simulink model "mcb_pmsm_foc_sensorless_f28379d1"  (R2026a)
settings: Solver=FixedStepDiscrete  StopTime=8  EnableMultiTasking=on
InitFcn:
  | mcb_pmsm_foc_sensorless_f28379d_datascript; mcb_pmsm_foc_sensorless_f28379d_kre_setup; mcb_pmsm_foc_sensorless_f28379d_spmsm_based_ipmsm_setup;
model workspace (MAT data in the model file):
  encoderResolution = 2000
  hallOffset = '0.5'
  indexOffset = 850
  polePairs = '4'
values from neighbouring files (symbols this model uses):
  acceleration = 10000/PU_System.N_base    [mcb_pmsm_foc_sensorless_f28379d_datascript.m]
  dataType = 'single'    [mcb_pmsm_foc_sensorless_f28379d_datascript.m]
  inverter = mcb.updateInverterParameters(pmsm,inverter,target)    [mcb_pmsm_foc_sensorless_f28379d_datascript.m]    (also in mcb_pmsm_foc_sensorless_f28379d_kre_setup.m = inverterSPMSM)
  KRE_Params_Vector = single([      KRE_OBSERVER_R_RATIO * motor.Rs;      pmsm.Ld;      pmsm.Lq;      pmsm.FluxPM;      Ts;      PU_System.V_base;      PU_System.I_base;      pmsm.N_base;      pmsm.p;      KRE_Profile.Alpha;      KRE_Profile.A;      KRE_Profile.Gamma;      KRE_Profile.SigmaEpsilon;      KRE_Profile.SpeedFilterHz])    [mcb_pmsm_foc_sensorless_f28379d_kre_setup.m]
  MAX_OL_NEG_SPD = -0.2    [mcb_pmsm_foc_sensorless_f28379d_datascript.m]
  MAX_OL_POS_SPD = 0.2    [mcb_pmsm_foc_sensorless_f28379d_datascript.m]
  MAX_OL_VD_LIMIT = 0.6    [mcb_pmsm_foc_sensorless_f28379d_datascript.m]
  MIN_CL_NEG_SPD = -0.15    [mcb_pmsm_foc_sensorless_f28379d_datascript.m]
  MIN_CL_POS_SPD = 0.15    [mcb_pmsm_foc_sensorless_f28379d_datascript.m]
  MIN_OL_VD_LIMIT = 0.15    [mcb_pmsm_foc_sensorless_f28379d_datascript.m]
  one_sec_tick = uint16(1/Ts_speed)    [mcb_pmsm_foc_sensorless_f28379d_datascript.m]
  PI_params = mcb.calcFOCGains(motor,Ts,Ts_speed,Base=PU_System,PositionObserver=EEMF,SLFeedbackPathDelay=EEMFSLDelay)    [mcb_pmsm_foc_sensorless_f28379d_datascript.m]    (also in mcb_pmsm_foc_sensorless_f28379d_kre_setup.m = PI_paramsSPMSM)
  pmsm = mcb.getPMSMParameters('Teknic2310P')    [mcb_pmsm_foc_sensorless_f28379d_datascript.m]    (also in mcb_pmsm_foc_sensorless_f28379d_kre_setup.m = pmsmSPMSM)
  PU_System = mcb.getPUSystemParameters(pmsm,inverter)    [mcb_pmsm_foc_sensorless_f28379d_datascript.m]    (also in mcb_pmsm_foc_sensorless_f28379d_kre_setup.m = PU_SystemSPMSM)
  RAMP_STEP_SIZE = 0.001    [mcb_pmsm_foc_sensorless_f28379d_datascript.m]
  Speed_openLoop_PU = 0.1    [mcb_pmsm_foc_sensorless_f28379d_datascript.m]
  target = mcb.getProcessorParameters('F28379D',PWM_frequency)    [mcb_pmsm_foc_sensorless_f28379d_datascript.m]
  Ts = T_pwm    (= 5e-05)    [mcb_pmsm_foc_sensorless_f28379d_datascript.m]
  Ts_motor = T_pwm/2    (= 2.5e-05)    [mcb_pmsm_foc_sensorless_f28379d_datascript.m]
  Ts_simulink = T_pwm/2    (= 2.5e-05)    [mcb_pmsm_foc_sensorless_f28379d_datascript.m]
  Ts_speed = 10*Ts    (= 0.0005)    [mcb_pmsm_foc_sensorless_f28379d_datascript.m]
  two_sec_tick = uint16(2/Ts_speed)    [mcb_pmsm_foc_sensorless_f28379d_datascript.m]
undefined symbols (not defined in the file or in its folder): bit, DiscIntNeverNeededParam, Down, GPTRIP1SEL, GPTRIP2SEL, TZ1, TZ2, Up
libraries: mcbcontrolslib x9, c2802xlib x7, mcbeeMathTransformLib x6, simulink x6, c280xlib x5, c2837xDlib x4, slpidlib x3, mcbpositiondecoderlib x3, mcbsensorlessestimatorlib x2, svdschedulerlib x2, svdutilitieslib x1, mcbplantlib x1
(part 1 of 3)
settings Model: ExtModeTrigDuration=8  Creator=The MathWorks, Inc.  LastModifiedBy=hzldx
settings OptimizationCC: DefaultUnderspecifiedDataType=single  OptimizeBlockIOStorage=off  BufferReuse=off  GlobalBufferReuse=off  ExpressionFolding=off  LocalBlockOutputs=off  InitFltsAndDblsToZero=on  NoFixptDivByZeroProtection=on  EfficientFloat2IntCast=on  EfficientMapNaN2IntZero=off  LifeSpan=Inf  MaxStackSize=1024  OptimizeDataStoreBuffers=off  BusAssignmentInplaceUpdate=off  DenormalBehavior=FlushToZero
settings DebuggingCC: ReadBeforeWriteMsg=DisableAll  WriteAfterWriteMsg=DisableAll  WriteAfterReadMsg=DisableAll  CheckSSInitialOutputMsg=off  InheritedTsInSrcMsg=none  MultiTaskDSMMsg=none  MultiTaskCondExecSysMsg=none  TasksWithSamePriorityMsg=none  SigSpecEnsureSampleTimeMsg=none  IntegerOverflowMsg=none  ParameterPrecisionLossMsg=none  SubsystemReferenceDiagnosticForUnitTest=warning  IntegerSaturationMsg=none
settings HardwareCC: ProdBitPerChar=16.0  ProdBitPerInt=16.0  ProdLargestAtomicInteger=Integer  ProdWordSize=16.0  ProdHWDeviceType=Texas Instruments->C2000  TargetBitPerChar=16.0  TargetBitPerInt=16.0  TargetBitPerPointer=16.0  TargetLargestAtomicInteger=Integer  TargetIntDivRoundTo=Zero  TargetEndianess=LittleEndian  TargetWordSize=16.0  TargetHWDeviceType=TI C2000
settings RTWCC: SystemTargetFile=ert.tlc  HardwareBoard=TI Delfino F28379D LaunchPad  GenerateReport=on  Toolchain=Texas Instruments Code Composer Studio (C2000)  IncludeHyperlinkInReport=on  LaunchReport=on  GenerateTraceInfo=on  GenerateTraceReport=on  GenerateTraceReportSl=on  GenerateTraceReportSf=on  GenerateTraceReportEml=on  Description=Embedded Coder
settings CodeAppCC: CustomSymbolStrType=$N$R$M  InternalIdentifier=Classic
settings ERTTargetCC: ExtModeStaticAllocSize=10000.0  MemSecPackage=tic2000demospkg  DynamicArrayContainerType=coder::array  CodeReplacementLibrary=TI C28x  MultiwordLength=2048.0
settings SimscapeCC: SimscapeNominalValues="[{\"value\":\"1\",\"unit\":\"A\"},{\"value\":\"1\",\"unit\":\"bar\"},{\"value\":\"1\",\"unit\":\"cm^2\"},{\"value\":\"1\",\"unit\":\"cm^3/s\"},{\"value\":\"1\",\"unit\":\"kJ/kg\"},{\"value\":\"1\",\"unit\":\"kW\"},{\"value\":\"1\",\"unit\":\"l\"},{\"value\":\"1\",\"unit\":\"N\"},{\"value\":\"1\",\"unit\":\"N*m\"},{\"value\":\"1\",\"unit\":\"V\"}]"  SimscapeLogType=none  SimscapeLogDataHistory=5000.0

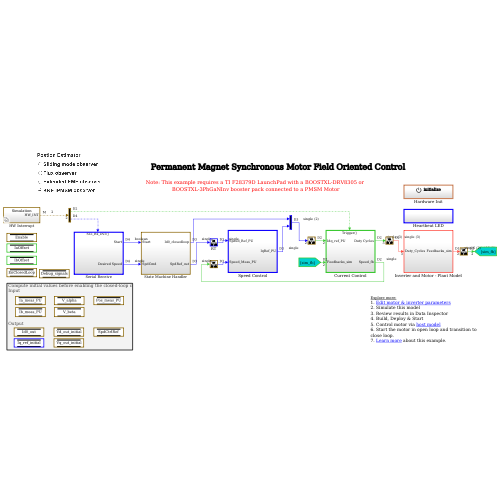
[thumbnail: Simulink's stored preview of the top-level diagram]
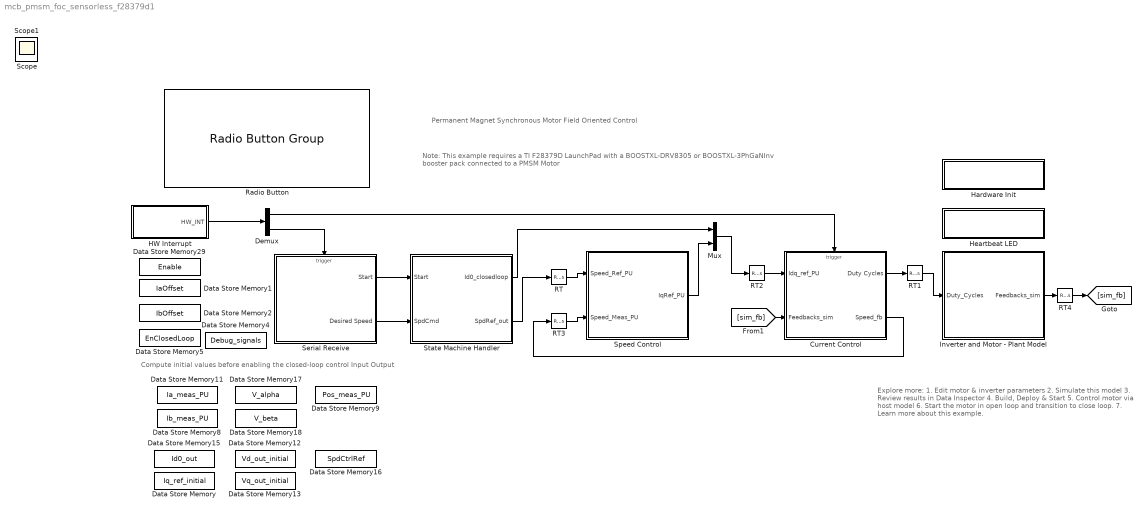
== system mcb_pmsm_foc_sensorless_f28379d1 ==
  note: Compute initial values before enabling the closed-loop control
      | Input
      |
      |
      |
      |
      |
      | Output
  note: Permanent Magnet Synchronous Motor Field Oriented Control
  note: Explore more:
      | 1. Edit motor & inverter parameters
      | 2. Simulate this model
      | 3. Review results in Data Inspector
      | 4. Build, Deploy & Start
      | 5. Control motor via host model
      | 6. Start the motor in open loop and transition to close loop.
      | 7. Learn more about this example.
  note: Note: This example requires a TI F28379D LaunchPad with a BOOSTXL-DRV8305 or
      | BOOSTXL-3PhGaNInv booster pack connected to a PMSM Motor
  Current Control : Subsystem
  Data Store Memory : DataStoreMemory  DataStoreName=Iq_ref_initial  WriteAfterWriteMsg=warning  ShowAdditionalParam=off  OutDataTypeStr=dataType
  Data Store Memory1 : DataStoreMemory  DataStoreName=IaOffset  InitialValue=inverter.CtSensAOffset  ShowAdditionalParam=off  OutDataTypeStr=uint16
  Data Store Memory11 : DataStoreMemory  DataStoreName=Ia_meas_PU  WriteAfterWriteMsg=warning  ShowAdditionalParam=off  OutDataTypeStr=dataType
  Data Store Memory12 : DataStoreMemory  DataStoreName=Vd_out_initial  WriteAfterWriteMsg=warning  ShowAdditionalParam=off  OutDataTypeStr=dataType
  Data Store Memory13 : DataStoreMemory  DataStoreName=Vq_out_initial  WriteAfterWriteMsg=warning  ShowAdditionalParam=off  OutDataTypeStr=dataType
  Data Store Memory15 : DataStoreMemory  DataStoreName=Id0_out  InitialValue=0.1  ShowAdditionalParam=off  OutDataTypeStr=dataType
  Data Store Memory16 : DataStoreMemory  DataStoreName=SpdCtrlRef  InitialValue=0.1  ShowAdditionalParam=off  OutDataTypeStr=dataType
  Data Store Memory17 : DataStoreMemory  DataStoreName=V_alpha  WriteAfterWriteMsg=warning  ShowAdditionalParam=off  OutDataTypeStr=dataType
  Data Store Memory18 : DataStoreMemory  DataStoreName=V_beta  WriteAfterWriteMsg=warning  ShowAdditionalParam=off  OutDataTypeStr=dataType
  Data Store Memory2 : DataStoreMemory  DataStoreName=IbOffset  InitialValue=inverter.CtSensBOffset  ShowAdditionalParam=off
  Data Store Memory29 : DataStoreMemory  DataStoreName=Enable  ShowAdditionalParam=off  OutDataTypeStr=boolean
  Data Store Memory4 : DataStoreMemory  DataStoreName=Debug_signals  InitialValue=5  ShowAdditionalParam=off  OutDataTypeStr=uint16
  Data Store Memory5 : DataStoreMemory  DataStoreName=EnClosedLoop  ShowAdditionalParam=off  OutDataTypeStr=boolean
  Data Store Memory8 : DataStoreMemory  DataStoreName=Ib_meas_PU  WriteAfterWriteMsg=warning  ShowAdditionalParam=off  OutDataTypeStr=dataType
  Data Store Memory9 : DataStoreMemory  DataStoreName=Pos_meas_PU  ShowAdditionalParam=off  OutDataTypeStr=dataType
  Demux : Demux  Outputs=2
  HW Interrupt : Subsystem  Variant=on  VariantControlMode=sim codegen switching
  Hardware Init : Subsystem  TreatAsAtomicUnit=on
  Heartbeat LED : Subsystem  TreatAsAtomicUnit=on
  Inverter and Motor - Plant Model : Subsystem
  Mux : Mux  Inputs=2
  RT : RateTransition  Deterministic=off  OutPortSampleTime=Ts_speed
  RT1 : RateTransition  Deterministic=off
  RT2 : RateTransition  Deterministic=off
  RT3 : RateTransition  Deterministic=off  OutPortSampleTime=Ts_speed
  RT4 : RateTransition  Deterministic=off
  Radio Button : RadioButtonGroup  LabelPosition=Hide  SelectedLabel=KRE IPMSM observer  ButtonGroupName=Postion Estimator
  Serial Receive : Subsystem  SystemSampleTime=1e-3
  Speed Control : Subsystem  Priority=50  TreatAsAtomicUnit=on  SystemSampleTime=Ts_speed
  State Machine Handler : Subsystem
  Scope : Scope
      settings: ActiveDisplayYMinimum=-0.125  ActiveDisplayYMaximum=1.125
  Scope1 : Scope
      settings: ActiveDisplayYMinimum=-0.125  ActiveDisplayYMaximum=1.125
  wires:
  RT3/1 -> Speed Control/2(Speed_Meas_PU)
  Inverter and Motor - Plant Model/1(Feedbacks_sim) -> RT4/1
  Demux/2 -> Serial Receive/Trigger
  RT/1 -> Speed Control/1(Speed_Ref_PU)
  HW Interrupt/1(HW_INT) -> Demux/1
  RT4/1 -> [sim_fb]
  RT1/1 -> Inverter and Motor - Plant Model/1(Duty_Cycles)
  Current Control/2(Speed_fb) -> RT3/1
  Demux/1 -> Current Control/Trigger
  [sim_fb] -> Current Control/2(Feedbacks_sim)
  Current Control/1(Duty Cycles) -> RT1/1
  RT2/1 -> Current Control/1(Idq_ref_PU)
  State Machine Handler/1(Id0_closedloop) -> Mux/1
  Serial Receive/1(Start) -> State Machine Handler/1(Start)
  State Machine Handler/2(SpdRef_out) -> RT/1
  Speed Control/1(IqRef_PU) -> Mux/2
  Mux/1 -> RT2/1
  Serial Receive/2(Desired Speed) -> State Machine Handler/2(SpdCmd)

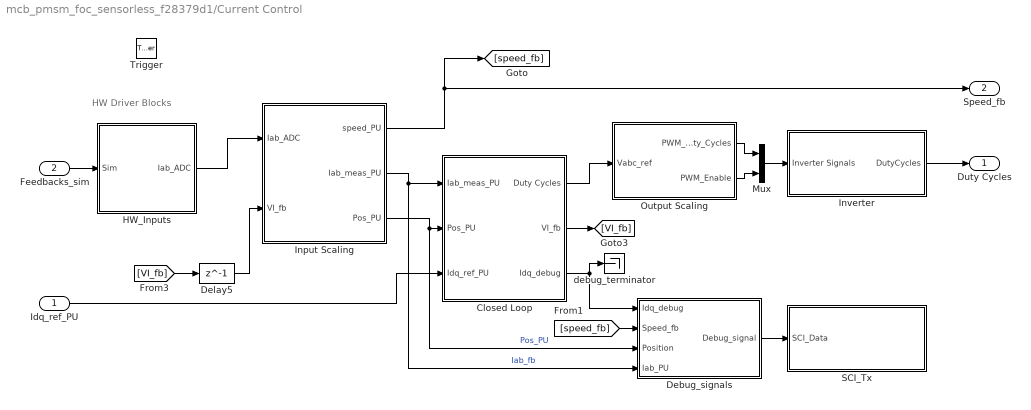
== system mcb_pmsm_foc_sensorless_f28379d1/Current Control ==
  note: HW Driver Blocks
  Idq_ref_PU : Inport
  Feedbacks_sim : Inport  Port=2
  Trigger : TriggerPort  TriggerType=function-call  VariantControl=Variant  PortDimensions=1
  Closed Loop : Subsystem
  Debug_signals : Subsystem
  Delay5 : Delay  DelayLength=1
  HW_Inputs : Subsystem  Variant=on  VariantControlMode=sim codegen switching
  Input Scaling : Subsystem
  Inverter : Subsystem  Variant=on  VariantControlMode=sim codegen switching
  Mux : Mux  Inputs=2
  Output Scaling : Subsystem
  SCI_Tx : Subsystem  Variant=on  VariantControlMode=sim codegen switching
  debug_terminator : Terminator
  Duty Cycles : Outport  InitialOutput=0  VectorParamsAs1DForOutWhenUnconnected=off
  Speed_fb : Outport  Port=2  InitialOutput=0  VectorParamsAs1DForOutWhenUnconnected=off
  wires:
  Closed Loop/1(Duty Cycles) -> Output Scaling/1(Vabc_ref)
  Input Scaling/3(Pos_PU) -> Debug_signals/3(Position), Closed Loop/2(Pos_PU)  "Pos_PU"
  Idq_ref_PU/1 -> Closed Loop/3(Idq_ref_PU)
  Input Scaling/2(Iab_meas_PU) -> Closed Loop/1(Iab_meas_PU), Debug_signals/4(Iab_PU)  "Iab_fb"
  Output Scaling/1(PWM_Duty_Cycles) -> Mux/1
  Mux/1 -> Inverter/1(Inverter Signals)
  Output Scaling/2(PWM_Enable) -> Mux/2
  Inverter/1(DutyCycles) -> Duty Cycles/1
  HW_Inputs/1(Iab_ADC) -> Input Scaling/1(Iab_ADC)
  Feedbacks_sim/1 -> HW_Inputs/1(Sim)
  Closed Loop/2(VI_fb) -> [VI_fb]
  [VI_fb] -> Delay5/1
  Input Scaling/1(speed_PU) -> [speed_fb], Speed_fb/1
  Closed Loop/3(Idq_debug) -> debug_terminator/1, Debug_signals/1(Idq_debug)
  [speed_fb] -> Debug_signals/2(Speed_fb)
  Debug_signals/1(Debug_signal) -> SCI_Tx/1(SCI_Data)
  Delay5/1 -> Input Scaling/2(VI_fb)

== system mcb_pmsm_foc_sensorless_f28379d1/HW Interrupt ==
  Code generation : Subsystem  VariantControl=(codegen)
  Simulation : Subsystem  VariantControl=(sim)
  HW_INT : Outport  OutputFunctionCall=on

== system mcb_pmsm_foc_sensorless_f28379d1/Hardware Init ==
  6PWM_Mode : Constant  Priority=1000  Value=0x3A16  OutDataTypeStr=uint16  SampleTime=-1
  ADC_Gain_Setting : Constant  Priority=1000  Value=inverter.SPI_Gain_Setting  OutDataTypeStr=uint16  SampleTime=-1
  Event Listener : EventListener  DisableCoverage=on  EventName=reset
  Mux : Mux  Inputs=2
  Variant Subsystem : Subsystem  Variant=on  VariantControlMode=sim codegen switching
  wires:
  6PWM_Mode/1 -> Mux/1
  ADC_Gain_Setting/1 -> Mux/2
  Mux/1 -> Variant Subsystem/1(In1)

== system mcb_pmsm_foc_sensorless_f28379d1/Heartbeat LED ==
  note: Heartbeat LED 1 Hz
  Heartbeat LED : Subsystem  Variant=on  VariantControlMode=sim codegen switching
  RED_LED : Constant  OutDataTypeStr=uint16  SampleTime=0.5
  wires:
  RED_LED/1 -> Heartbeat LED/1(In1)

== system mcb_pmsm_foc_sensorless_f28379d1/Inverter and Motor - Plant Model ==
  Duty_Cycles : Inport
  Codegeneration : Subsystem
  Simulation : Subsystem
  Variant Sink : VariantSink  VariantControlMode=sim codegen switching  VariantControls={(codegen), (sim)}
  Variant Source1 : VariantSource  VariantControlMode=sim codegen switching  VariantControls={(codegen), (sim)}
  Feedbacks_sim : Outport  VectorParamsAs1DForOutWhenUnconnected=off
  wires:
  Duty_Cycles/1 -> Variant Sink/1
  Simulation/1(Feedbacks) -> Variant Source1/2
  Variant Sink/2 -> Simulation/1(Duty_Cycles)
  Variant Source1/1 -> Feedbacks_sim/1
  Variant Sink/1 -> Codegeneration/1(Duty_Cycles)
  Codegeneration/1(Feedbacks) -> Variant Source1/1

== system mcb_pmsm_foc_sensorless_f28379d1/Serial Receive ==
  SCI_Rx_INT : TriggerPort  TriggerType=function-call  VariantControl=Variant
  Data Store Write2 : DataStoreWrite  DataStoreName=Debug_signals  IndexOptions=Index vector (dialog)  Indices=1  OutputSizes=1
  Data_Conditioning_Rx : Subsystem  Variant=on
  SCI_Rx : Subsystem  Variant=on  VariantControlMode=sim codegen switching
  unParse : Subsystem
  Start : Outport  VectorParamsAs1DForOutWhenUnconnected=off
  Desired Speed : Outport  Port=2  VectorParamsAs1DForOutWhenUnconnected=off
  wires:
  unParse/2(Debug_signals) -> Data Store Write2/1
  unParse/1(Enable_PWM) -> Start/1
  Data_Conditioning_Rx/2(Out2) -> unParse/1(Data)
  Data_Conditioning_Rx/1(Desired Speed) -> Desired Speed/1
  SCI_Rx/1(Data) -> Data_Conditioning_Rx/1(In1)

== system mcb_pmsm_foc_sensorless_f28379d1/Speed Control ==
  Speed_Ref_PU : Inport
  Speed_Meas_PU : Inport  Port=2
  PI_Controller_Speed : Subsystem
  SlewRate : Subsystem
  IqRef_PU : Outport  VectorParamsAs1DForOutWhenUnconnected=off
  wires:
  Speed_Meas_PU/1 -> PI_Controller_Speed/2(N_fb)  "Speed_fb"
  SlewRate/1(N_ref) -> PI_Controller_Speed/1(N_ref)  "Spd_filt"
  Speed_Ref_PU/1 -> SlewRate/1(Speed_Ref)  "Speed_Ref"
  PI_Controller_Speed/1(Iq_ref) -> IqRef_PU/1

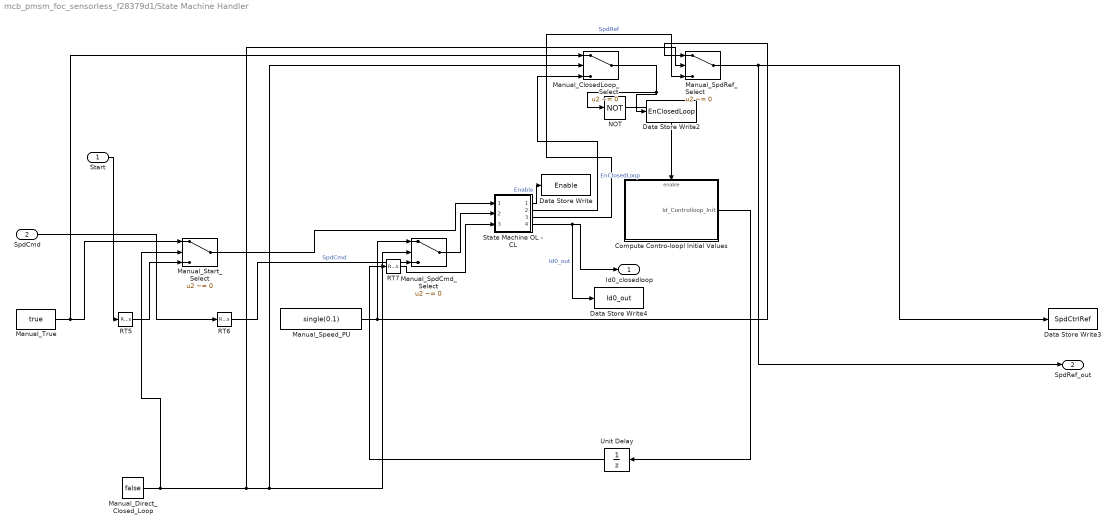
== system mcb_pmsm_foc_sensorless_f28379d1/State Machine Handler ==
  Start : Inport
  SpdCmd : Inport  Port=2
  Compute Contro-loopl Initial Values : Subsystem
  Data Store Write : DataStoreWrite  DataStoreName=Enable  IndexOptions=Index vector (dialog)  Indices=1  OutputSizes=1
  Data Store Write2 : DataStoreWrite  DataStoreName=EnClosedLoop  IndexOptions=Index vector (dialog)  Indices=1  OutputSizes=1
  Data Store Write3 : DataStoreWrite  DataStoreName=SpdCtrlRef  IndexOptions=Index vector (dialog)  Indices=1  OutputSizes=1
  Data Store Write4 : DataStoreWrite  DataStoreName=Id0_out  IndexOptions=Index vector (dialog)  Indices=1  OutputSizes=1
  Manual_ClosedLoop_Select : Switch  Criteria=u2 ~= 0  Threshold=0.5  SaturateOnIntegerOverflow=off  InputSameDT=off
  Manual_Direct_Closed_Loop : Constant  Value=false  OutDataTypeStr=boolean  SampleTime=-1
  Manual_SpdCmd_Select : Switch  Criteria=u2 ~= 0  Threshold=0.5  SaturateOnIntegerOverflow=off  InputSameDT=off
  Manual_SpdRef_Select : Switch  Criteria=u2 ~= 0  Threshold=0.5  SaturateOnIntegerOverflow=off  InputSameDT=off
  Manual_Speed_PU : Constant  Value=single(0.1)  SampleTime=-1
  Manual_Start_Select : Switch  Criteria=u2 ~= 0  Threshold=0.5  SaturateOnIntegerOverflow=off  InputSameDT=off
  Manual_True : Constant  Value=true  OutDataTypeStr=boolean  SampleTime=-1
  NOT : Logic  Operator=NOT  IconShape=distinctive  AllPortsSameDT=off  OutDataTypeStr=boolean
  RT5 : RateTransition  Deterministic=off  OutPortSampleTime=Ts_speed
  RT6 : RateTransition  Deterministic=off  OutPortSampleTime=Ts_speed
  RT7 : RateTransition  Deterministic=off  OutPortSampleTime=Ts_speed
  State Machine OL - CL : Stateflow chart  Priority=10  TreatAsAtomicUnit=on  SystemSampleTime=Ts_speed
  Unit Delay : UnitDelay  SampleTime=-1
  Id0_closedloop : Outport
  SpdRef_out : Outport  Port=2
  wires:
  NOT/1 -> Compute Contro-loopl Initial Values/Enable
  Unit Delay/1 -> RT7/1
  Compute Contro-loopl Initial Values/1(Id_Controlloop_Init) -> Unit Delay/1
  State Machine OL - CL/3(SpdRef) -> Manual_SpdRef_Select/3  "SpdRef"
  State Machine OL - CL/2(EnClosedLoop) -> Manual_ClosedLoop_Select/3  "EnClosedLoop"
  RT6/1 -> Manual_SpdCmd_Select/3  "SpdCmd"
  RT5/1 -> Manual_Start_Select/3
  Manual_SpdRef_Select/1 -> Data Store Write3/1, SpdRef_out/1
  Manual_ClosedLoop_Select/1 -> Data Store Write2/1, NOT/1
  Manual_SpdCmd_Select/1 -> State Machine OL - CL/2(SpdCmd)
  Manual_Speed_PU/1 -> Manual_SpdRef_Select/1, Manual_SpdCmd_Select/1
  Manual_Start_Select/1 -> State Machine OL - CL/1(Start)
  Manual_True/1 -> Manual_ClosedLoop_Select/1, Manual_Start_Select/1
  Manual_Direct_Closed_Loop/1 -> Manual_ClosedLoop_Select/2, Manual_SpdCmd_Select/2, Manual_SpdRef_Select/2, Manual_Start_Select/2
  RT7/1 -> State Machine OL - CL/3(Id0_in)
  SpdCmd/1 -> RT6/1
  State Machine OL - CL/1(Enable) -> Data Store Write/1  "Enable"
  Start/1 -> RT5/1
  State Machine OL - CL/4(Id0_out) -> Data Store Write4/1, Id0_closedloop/1  "Id0_out"

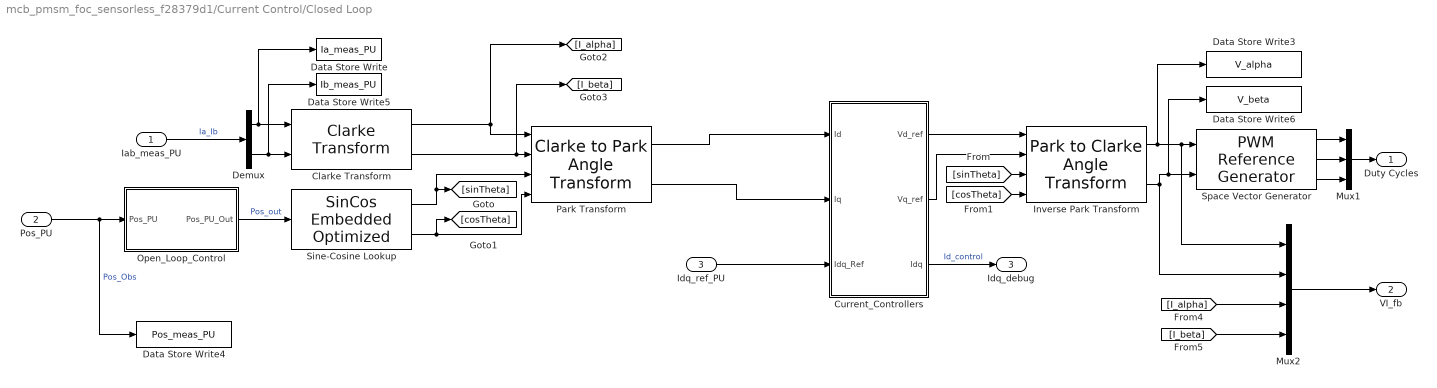
== system mcb_pmsm_foc_sensorless_f28379d1/Current Control/Closed Loop ==
  Iab_meas_PU : Inport
  Pos_PU : Inport  Port=2
  Idq_ref_PU : Inport  Port=3
  Clarke Transform : mcbeeMathTransformLib/Clarke Transform  VariantControl=Variant2  PowerInvariant=off  UseWithEmbedded=on  PhaseInput=Two inputs
  Current_Controllers : Subsystem
  Data Store Write : DataStoreWrite  DataStoreName=Ia_meas_PU  IndexOptions=Index vector (dialog)  Indices=1  OutputSizes=1
  Data Store Write3 : DataStoreWrite  DataStoreName=V_alpha  IndexOptions=Index vector (dialog)  Indices=1  OutputSizes=1
  Data Store Write4 : DataStoreWrite  DataStoreName=Pos_meas_PU  IndexOptions=Index vector (dialog)  Indices=1  OutputSizes=1
  Data Store Write5 : DataStoreWrite  DataStoreName=Ib_meas_PU  IndexOptions=Index vector (dialog)  Indices=1  OutputSizes=1
  Data Store Write6 : DataStoreWrite  DataStoreName=V_beta  IndexOptions=Index vector (dialog)  Indices=1  OutputSizes=1
  Demux : Demux  Outputs=2
  Inverse Park Transform : mcbeeMathTransformLib/Park to Clarke Angle Transform  AxisAlignment=D-axis  UseWithEmbedded=on  PhaseInput=Two inputs  ThetaInput=Sine and Cosine electrical position  AngleInput=Per-unit  N_points=1024
  Mux1 : Mux  Inputs=3
  Mux2 : Mux
  Open_Loop_Control : Subsystem
  Park Transform : mcbeeMathTransformLib/Clarke to Park Angle Transform  AxisAlignment=D-axis  UseWithEmbedded=on  PhaseInput=Two inputs  ThetaInput=Sine and Cosine electrical position  AngleInput=Per-unit  N_points=1024
  Sine-Cosine Lookup : mcbcontrolslib/SinCos Embedded Optimized  LabelModeActiveChoice=MCB_Sin  OptforProc=off  OptLevelPop=Disabled  ApproximationMethod=None  UserApproxMethod=Lookup  ApproxStatus=None  ThetaDataType=single  CopyThetaDataType=single  InterpMethod=Linear point-slope  NumberOfDataPoints=16  NumberOfIterations=11  RemoveProtectionAgainstOutOfRangeInput=off  TableDataTypeStr=Inherit: Inherit via input  AngleInput=Per-unit  CopyAngleInput=Per-unit  N_points=1024  CopyN_points=1024  Datatype=single  CopyTableDatatype=single  DatatypeInput=Inherit from input  IsPrevStrictOpt=0  IsPrevLUTForced=0
  Space Vector Generator : mcbcontrolslib/PWM Reference Generator  modType=SVM: space vector modulation  inSignal=Valphabeta  expandVoltageInput=on  inputUnits=Per-unit  LimitModulation=off  enableVoltage=on  enableModulationSignal=off  enableDutyCycle=off  expandVoltageOutput=on
  Duty Cycles : Outport  VectorParamsAs1DForOutWhenUnconnected=off
  VI_fb : Outport  Port=2  VectorParamsAs1DForOutWhenUnconnected=off
  Idq_debug : Outport  Port=3  VectorParamsAs1DForOutWhenUnconnected=off
  wires:
  Current_Controllers/1(Vd_ref) -> Inverse Park Transform/1
  [cosTheta] -> Inverse Park Transform/4
  [I_beta] -> Mux2/4
  Inverse Park Transform/2 -> Mux2/2, Data Store Write6/1, Space Vector Generator/2
  Inverse Park Transform/1 -> Data Store Write3/1, Mux2/1, Space Vector Generator/1
  [sinTheta] -> Inverse Park Transform/3
  Mux2/1 -> VI_fb/1
  Clarke Transform/1 -> Park Transform/1, [I_alpha]
  Current_Controllers/2(Vq_ref) -> Inverse Park Transform/2
  Clarke Transform/2 -> [I_beta], Park Transform/2
  [I_alpha] -> Mux2/3
  Space Vector Generator/1 -> Mux1/1
  Space Vector Generator/3 -> Mux1/3
  Mux1/1 -> Duty Cycles/1
  Space Vector Generator/2 -> Mux1/2
  Park Transform/1 -> Current_Controllers/1(Id)
  Park Transform/2 -> Current_Controllers/2(Iq)
  Demux/1 -> Data Store Write/1, Clarke Transform/1
  Demux/2 -> Data Store Write5/1, Clarke Transform/2
  Iab_meas_PU/1 -> Demux/1  "Ia_Ib"
  Idq_ref_PU/1 -> Current_Controllers/3(Idq_Ref)
  Pos_PU/1 -> Data Store Write4/1, Open_Loop_Control/1(Pos_PU)  "Pos_Obs"
  Current_Controllers/3(Idq) -> Idq_debug/1  "Id_control"
  Open_Loop_Control/1(Pos_PU_Out) -> Sine-Cosine Lookup/1  "Pos_out"
  Sine-Cosine Lookup/1 -> Park Transform/3, [sinTheta]
  Sine-Cosine Lookup/2 -> Park Transform/4, [cosTheta]

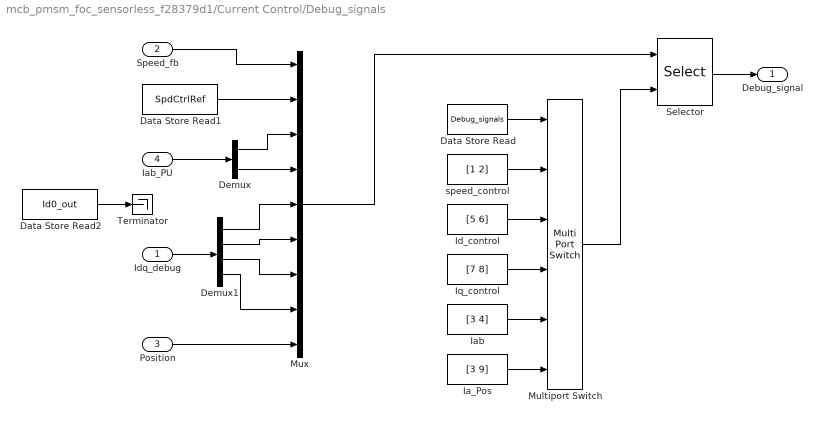
== system mcb_pmsm_foc_sensorless_f28379d1/Current Control/Debug_signals ==
  Idq_debug : Inport
  Speed_fb : Inport  Port=2
  Position : Inport  Port=3
  Iab_PU : Inport  Port=4
  Data Store Read : DataStoreRead  DataStoreName=Debug_signals  IndexOptions=Index vector (dialog)  Indices=1  OutputSizes=1
  Data Store Read1 : DataStoreRead  DataStoreName=SpdCtrlRef  IndexOptions=Index vector (dialog)  Indices=1  OutputSizes=1
  Data Store Read2 : DataStoreRead  DataStoreName=Id0_out  IndexOptions=Index vector (dialog)  Indices=1  OutputSizes=1
  Demux : Demux  Outputs=2
  Demux1 : Demux
  Ia_Pos : Constant  Value=[3 9]  OutDataTypeStr=uint16  SampleTime=-1
  Iab : Constant  Value=[3 4]  OutDataTypeStr=uint16  SampleTime=-1
  Id_control : Constant  Value=[5 6]  OutDataTypeStr=uint16  SampleTime=-1
  Iq_control : Constant  Value=[7 8]  OutDataTypeStr=uint16  SampleTime=-1
  Multiport Switch : MultiPortSwitch  Inputs=5  DiagnosticForDefault=Warning  OutDataTypeStr=uint16  RndMeth=Simplest  SaturateOnIntegerOverflow=off  InputSameDT=off
  Mux : Mux  Inputs=9
  Selector : Selector  InputPortWidth=9  IndexOptions=Index vector (port)  Indices=[1 3]  OutputSizes=1
  Terminator : Terminator
  speed_control : Constant  Value=[1 2]  OutDataTypeStr=uint16  SampleTime=-1
  Debug_signal : Outport
  wires:
  speed_control/1 -> Multiport Switch/2
  Id_control/1 -> Multiport Switch/3
  Iq_control/1 -> Multiport Switch/4
  Iab/1 -> Multiport Switch/5
  Ia_Pos/1 -> Multiport Switch/6
  Multiport Switch/1 -> Selector/2
  Data Store Read/1 -> Multiport Switch/1
  Selector/1 -> Debug_signal/1
  Data Store Read1/1 -> Mux/2
  Iab_PU/1 -> Demux/1
  Demux/1 -> Mux/3
  Demux/2 -> Mux/4
  Demux1/3 -> Mux/7
  Idq_debug/1 -> Demux1/1
  Mux/1 -> Selector/1
  Speed_fb/1 -> Mux/1
  Position/1 -> Mux/9
  Demux1/2 -> Mux/6
  Demux1/4 -> Mux/8
  Demux1/1 -> Mux/5
  Data Store Read2/1 -> Terminator/1

== system mcb_pmsm_foc_sensorless_f28379d1/Current Control/HW_Inputs ==
  Sim : Inport
  Sensor Driver Blocks (codegen) : Subsystem  VariantControl=(codegen)
  Sensor Driver Blocks (sim) : Subsystem  VariantControl=(sim)
  Iab_ADC : Outport

== system mcb_pmsm_foc_sensorless_f28379d1/Current Control/Input Scaling ==
  note: Current Measurements
  note: Position & Speed Measurements
  Iab_ADC : Inport
  VI_fb : Inport  Port=2
  Calculate Phase Currents : Subsystem
  Calculate position and speed : Subsystem
  speed_PU : Outport
  Iab_meas_PU : Outport  Port=2
  Pos_PU : Outport  Port=3
  wires:
  Calculate Phase Currents/1(Iab_meas_PU) -> Iab_meas_PU/1
  Iab_ADC/1 -> Calculate Phase Currents/1(Iab_ADC)
  Calculate position and speed/2(Pos_PU) -> Pos_PU/1
  Calculate position and speed/1(speed_PU) -> speed_PU/1
  VI_fb/1 -> Calculate position and speed/1(VI_fb)

== system mcb_pmsm_foc_sensorless_f28379d1/Current Control/Inverter ==
  Inverter Signals : Inport
  Code Generation : Subsystem  VariantControl=(codegen)
  Simulation : Subsystem  VariantControl=(sim)
  DutyCycles : Outport  VectorParamsAs1DForOutWhenUnconnected=off

== system mcb_pmsm_foc_sensorless_f28379d1/Current Control/Output Scaling ==
  Vabc_ref : Inport
  Constant : Constant  Value=0.5  OutDataTypeStr=dataType  SampleTime=-1
  Data Type Conversion : DataTypeConversion  OutDataTypeStr=dataType  SaturateOnIntegerOverflow=off  RndMeth=Floor
  Enable : DataStoreRead  DataStoreName=Enable  IndexOptions=Index vector (dialog)  Indices=1  OutputSizes=1
  One_by_Two : Gain  Gain=0.5  RndMeth=Simplest  OutDataTypeStr=Inherit: Same as input
  Sum : Sum  Inputs=|++
  PWM_Duty_Cycles : Outport
  PWM_Enable : Outport  Port=2
  wires:
  Constant/1 -> Sum/2
  Vabc_ref/1 -> One_by_Two/1
  Sum/1 -> PWM_Duty_Cycles/1  "PWM_Duty_Cycles"
  Enable/1 -> Data Type Conversion/1
  One_by_Two/1 -> Sum/1
  Data Type Conversion/1 -> PWM_Enable/1

== system mcb_pmsm_foc_sensorless_f28379d1/Current Control/SCI_Tx ==
  SCI_Data : Inport
  Code Generation : Subsystem  VariantControl=(codegen)
  Simulation : Subsystem  VariantControl=(sim)

== system mcb_pmsm_foc_sensorless_f28379d1/HW Interrupt/Code generation ==
  HWI_ADCB1_INT : svdschedulerlib/Hardware Interrupt v2  ISRGroup=ADC - Analog to Digital Converter  ISRName=ADCA1_INT  ISRNumber=32  NumEventsToServe=1  EventsList={'on','EOC event','1';'off','Overflow event','2';'off','Custom event','3'}  SelectedEvents={'event1'}  TaskPriority=30  DisablePreemption=on  ClearInterruptFlagsAtEndOfEvent=on  InterruptDefinitionFile=$(TARGET_ROOT)/registry/interrupts/F2837xS_interrupts.xml  HardwareBoard=F2837x  EnableSimPort=off
      settings: LibrarySourceBlock=c2000lib/Scheduling/Hardware Interrupt
  HWI_SCIA_RX_INT : svdschedulerlib/Hardware Interrupt v2  ISRGroup=ADC - Analog to Digital Converter  ISRName=ADCA1_INT  ISRNumber=32  NumEventsToServe=1  EventsList={'on','EOC event','1';'off','Overflow event','2';'off','Custom event','3'}  SelectedEvents={'event1'}  TaskPriority=50  DisablePreemption=off  ClearInterruptFlagsAtEndOfEvent=on  InterruptDefinitionFile=$(TARGET_ROOT)/registry/interrupts/F2837xS_interrupts.xml  HardwareBoard=F2837x  EnableSimPort=off
      settings: LibrarySourceBlock=c2000lib/Scheduling/Hardware Interrupt
  Mux : Mux  Inputs=2
  HW_INT : Outport
  wires:
  Mux/1 -> HW_INT/1
  HWI_ADCB1_INT/1 -> Mux/1
  HWI_SCIA_RX_INT/1 -> Mux/2

== system mcb_pmsm_foc_sensorless_f28379d1/HW Interrupt/Simulation ==
  ADCINT1 : FunctionCallGenerator  SampleTime=Ts
  Mux : Mux  Inputs=2
  SCI_Rx_INT : FunctionCallGenerator  SampleTime=0.1
  HW_INT : Outport
  wires:
  SCI_Rx_INT/1 -> Mux/2
  ADCINT1/1 -> Mux/1
  Mux/1 -> HW_INT/1

== system mcb_pmsm_foc_sensorless_f28379d1/Hardware Init/Variant Subsystem ==
  In1 : Inport
  Code Generation : Subsystem  VariantControl=(codegen)
  Simulation : Subsystem  VariantControl=(sim)

== system mcb_pmsm_foc_sensorless_f28379d1/Heartbeat LED/Heartbeat LED ==
  In1 : Inport
  Code generation : Subsystem  VariantControl=(codegen)
  Simulation : Subsystem  VariantControl=(sim)

== system mcb_pmsm_foc_sensorless_f28379d1/Inverter and Motor - Plant Model/Codegeneration ==
  Duty_Cycles : Inport
  Ground : Ground
  Terminator : Terminator
  Feedbacks : Outport  VectorParamsAs1DForOutWhenUnconnected=off
  wires:
  Duty_Cycles/1 -> Terminator/1
  Ground/1 -> Feedbacks/1

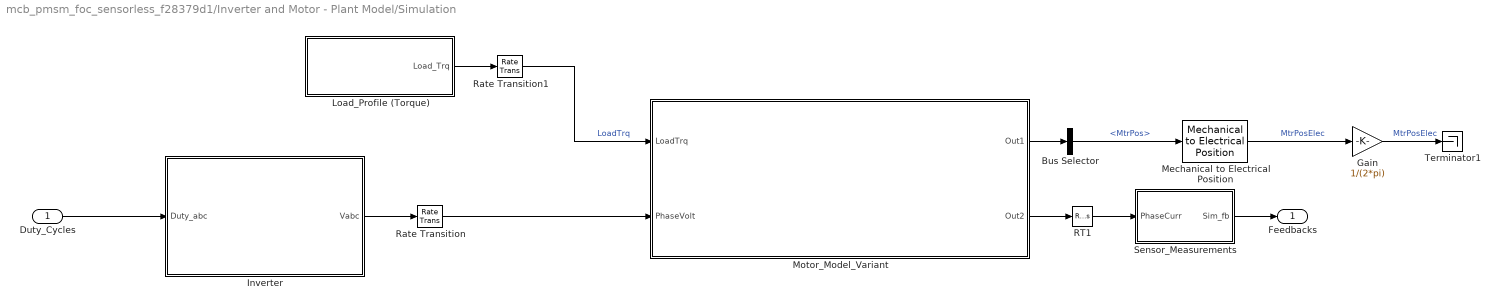
== system mcb_pmsm_foc_sensorless_f28379d1/Inverter and Motor - Plant Model/Simulation ==
  Duty_Cycles : Inport
  Bus Selector : BusSelector  OutputSignals=MtrPos
  Gain : Gain  Gain=1/(2*pi)  OutDataTypeStr=Inherit: Same as input
  Inverter : Subsystem
  Load_Profile (Torque) : Subsystem
  Mechanical to Electrical Position : mcbpositiondecoderlib/Mechanical to Electrical Position  PolePairsInputType=Specify via dialog  NrPP=pmsm.p  selectedRange=Radians  MechOfstInputType=Specify via dialog  mechOffsetIn=0  maxAngleIn=2*pi  InputDataType=single  VariantSelect=floating-point
  Motor_Model_Variant : Subsystem
  RT1 : RateTransition  Deterministic=off  OutPortSampleTime=Ts_simulink
  Rate Transition : RateTransition  Deterministic=off  OutPortSampleTime=Ts_motor
  Rate Transition1 : RateTransition  Deterministic=off  OutPortSampleTime=Ts_motor
  Sensor_Measurements : Subsystem
  Terminator1 : Terminator
  Feedbacks : Outport  VectorParamsAs1DForOutWhenUnconnected=off
  wires:
  Sensor_Measurements/1(Sim_fb) -> Feedbacks/1
  Mechanical to Electrical Position/1 -> Gain/1  "MtrPosElec"
  Bus Selector/1 -> Mechanical to Electrical Position/1  "<MtrPos>"
  Gain/1 -> Terminator1/1  "MtrPosElec"
  Inverter/1(Vabc) -> Rate Transition/1
  Load_Profile (Torque)/1(Load_Trq) -> Rate Transition1/1
  RT1/1 -> Sensor_Measurements/1(PhaseCurr)
  Duty_Cycles/1 -> Inverter/1(Duty_abc)
  Rate Transition1/1 -> Motor_Model_Variant/1(LoadTrq)  "LoadTrq"
  Rate Transition/1 -> Motor_Model_Variant/2(PhaseVolt)
  Motor_Model_Variant/1(Out1) -> Bus Selector/1
  Motor_Model_Variant/2(Out2) -> RT1/1

== system mcb_pmsm_foc_sensorless_f28379d1/Serial Receive/Data_Conditioning_Rx ==
  In1 : Inport
  Data_Type_Fixed_Point : Subsystem  VariantControl=~isequal(dataType, 'single')
  Data_Type_Float : Subsystem  VariantControl=isequal(dataType, 'single')
  Desired Speed : Outport
  Out2 : Outport  Port=2

== system mcb_pmsm_foc_sensorless_f28379d1/Serial Receive/SCI_Rx ==
  Code Generation : Subsystem  Variant=on  VariantControl=(codegen)
  Simulation : Subsystem  VariantControl=(sim)
  Data : Outport

== system mcb_pmsm_foc_sensorless_f28379d1/Serial Receive/unParse ==
  Data : Inport
  Bitwise Operator : simulink/Logic and Bit Operations/Bitwise Operator  logicop=AND  UseBitMask=on  BitMask=hex2dec('0001')  BitMaskRealWorld=Stored Integer
  Bitwise Operator1 : simulink/Logic and Bit Operations/Bitwise Operator  logicop=AND  UseBitMask=on  BitMask=hex2dec('00F0')  BitMaskRealWorld=Stored Integer
  Data Type Conversion3 : DataTypeConversion  OutDataTypeStr=boolean  RndMeth=Simplest  SaturateOnIntegerOverflow=off
  Data Type Conversion4 : DataTypeConversion  OutDataTypeStr=uint16  RndMeth=Simplest  SaturateOnIntegerOverflow=off
  Shift Arithmetic1 : ArithShift  BitShiftNumber=4
  Enable_PWM : Outport
  Debug_signals : Outport  Port=2
  wires:
  Bitwise Operator1/1 -> Shift Arithmetic1/1
  Data/1 -> Bitwise Operator/1, Bitwise Operator1/1
  Bitwise Operator/1 -> Data Type Conversion3/1
  Data Type Conversion4/1 -> Debug_signals/1
  Shift Arithmetic1/1 -> Data Type Conversion4/1
  Data Type Conversion3/1 -> Enable_PWM/1

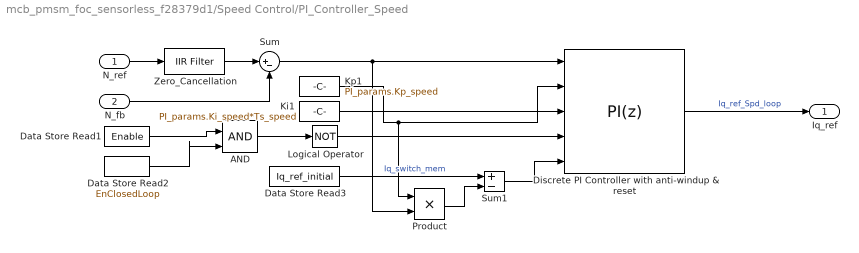
== system mcb_pmsm_foc_sensorless_f28379d1/Speed Control/PI_Controller_Speed ==
  N_ref : Inport
  N_fb : Inport  Port=2
  AND : Logic  IconShape=distinctive  AllPortsSameDT=off  OutDataTypeStr=boolean
  Data Store Read2 : DataStoreRead  DataStoreName=EnClosedLoop  IndexOptions=Index vector (dialog)  Indices=1  OutputSizes=1
  Data Store Read3 : DataStoreRead  DataStoreName=Iq_ref_initial  IndexOptions=Index vector (dialog)  Indices=1  OutputSizes=1
  Data Store Read1 : DataStoreRead  DataStoreName=Enable  IndexOptions=Index vector (dialog)  Indices=1  OutputSizes=1
  Discrete PI Controller with anti-windup & reset : slpidlib/PID Controller  Controller=PI  Form=Parallel  TimeDomain=Discrete-time  UseExternalTs=off  SampleTime=-1  IntegratorMethod=Forward Euler  FilterMethod=Forward Euler  ControllerParametersSource=external  P=1  I=1  UseKiTs=on  D=0  UseExternalDerivativeSource=off  N=100  UseFilter=on  TunerSelectOption=Transfer Function Based (PID Tuner App)  InitialConditionSource=external  InitialConditionForIntegrator=0  InitialConditionForFilter=0  DifferentiatorICPrevScaledInput=0  ExternalReset=level  TrackingMode=off  Kt=1  LimitOutput=on  SatLimitsSource=internal  UpperSaturationLimit=1  LowerSaturationLimit=-1  LinearizeAsGain=on  AntiWindupMode=clamping  Kb=1  LimitIntegrator=off  UpperIntegratorSaturationLimit=inf  LowerIntegratorSaturationLimit=-inf  RndMeth=Simplest  POutMin=[]  POutMax=[]  IOutMin=[]  IOutMax=[]  DOutMin=[]  DOutMax=[]  NOutMin=[]  NOutMax=[]  SumOutMin=[]  SumOutMax=[]  SaturationOutDataTypeStr=Inherit: Inherit via back propagation  SaturationOutMin=[]  SaturationOutMax=[]  PParamMin=[]  PParamMax=[]  IParamMin=[]  IParamMax=[]  DParamMin=[]  DParamMax=[]  NParamMin=[]  NParamMax=[]  KbParamMin=[]  KbParamMax=[]  KtParamMin=[]  KtParamMax=[]  KbOutMin=[]  KbOutMax=[]  KtOutMin=[]  KtOutMax=[]  IntegratorOutMin=[]  IntegratorOutMax=[]  FilterOutMin=[]  FilterOutMax=[]  SumI1OutMin=[]  SumI1OutMax=[]  SumI2OutMin=[]  SumI2OutMax=[]  SumI3OutMin=[]  SumI3OutMax=[]  SumI4OutMin=[]  SumI4OutMax=[]  SumDOutMin=[]  SumDOutMax=[]  DifferentiatorOutMin=[]  DifferentiatorOutMax=[]  FilterDiffOutCoefMin=[]  FilterDiffOutCoefMax=[]  ReciprocalOutMin=[]  ReciprocalOutMax=[]  SumDenOutMin=[]  SumDenOutMax=[]  SumNumOutMin=[]  SumNumOutMax=[]  DivideOutMin=[]  DivideOutMax=[]  UdiffTsProdOutMin=[]  UdiffTsProdOutMax=[]  NTsProdOutMin=[]  NTsProdOutMax=[]  UintegralTsProdOutMin=[]  UintegralTsProdOutMax=[]  UngainTsProdOutMin=[]  UngainTsProdOutMax=[]  ClampingZeroOutDataTypeStr=Inherit: Inherit via back propagation  ClampingZeroOutMin=[]  ClampingZeroOutMax=[]  FilterDenConstantOutDataTypeStr=Inherit: Inherit via back propagation  FilterDenConstantOutMin=[]  FilterDenConstantOutMax=[]  PCopyOutDataTypeStr=Inherit: Inherit via back propagation  PCopyOutMin=[]  PCopyOutMax=[]  NCopyOutDataTypeStr=Inherit: Inherit via back propagation  NCopyOutMin=[]  NCopyOutMax=[]  IntegratorContinuousStateAttributes=''  IntegratorStateMustResolveToSignalObject=off  IntegratorRTWStateStorageClass=Auto  FilterContinuousStateAttributes=''  FilterStateMustResolveToSignalObject=off  FilterRTWStateStorageClass=Auto  ParallelPVariant=ExternalParameters  IdealPVariant=Disabled  IVariant=ExternalParameters  DVariant=Disabled  IntegratorVariant=Discrete  SatVariant=Enabled  AWVariant=DiscClampingParallel  PCopyVariant=Disabled  TRVariant=Disabled  FdbkBlocksVariant=Forward  IdealPFdbkVariant=Disabled  SatFdbkVariant=Disabled  DerivativeFilterVariant=Disabled  NVariant=Disabled  NCopyVariant=Disabled_SignalSpec  FilterICVariant=Disabled  IntegratorICVariant=ExternalICs  ExternalResetVariant=ExternalReset  TRSumVariant=Passthrough  SumFdbkVariant=Disabled  SumVariant=Sum_PI  TsampFilterVariant=InternalTs  TsampNgainVariant=Passthrough  TsampIntegralVariant=Disabled_SignalSpec  ExternalSaturationOutDataTypeStr=Inherit: Same as second input  DerivativeSourceVariant=Disabled  PreIntVariant=InternalPreInt
      settings: LibrarySourceBlock=mcbcontrolslib/PI Controller
  Ki1 : Constant  Value=PI_params.Ki_speed*Ts_speed  OutDataTypeStr=dataType  SampleTime=-1
  Kp1 : Constant  Value=PI_params.Kp_speed  OutDataTypeStr=dataType  SampleTime=-1
  Logical Operator : Logic  Operator=NOT  IconShape=distinctive  AllPortsSameDT=off  OutDataTypeStr=boolean
  Product : Product  OutDataTypeStr=Inherit: Same as first input
  Sum : Sum  Inputs=|+-  OutDataTypeStr=Inherit: Same as first input
  Sum1 : Sum  Inputs=+-  OutDataTypeStr=Inherit: Same as first input
  Zero_Cancellation : mcbcontrolslib/IIR Filter  VariantControl=Low Pass Filter  VariantSelect=Low-pass  FilterConstantInputType=Specify via dialog  Filter_constant=0.01*(Ts_speed/Ts)  InitialOutput=Specify via dialog  InitialOutputValue=0  ExternalReset=none  advancedSettings=off  Ts=50e-6  cutOff_freq=353.6777
  Iq_ref : Outport  VectorParamsAs1DForOutWhenUnconnected=off
  wires:
  Discrete PI Controller with anti-windup & reset/1 -> Iq_ref/1  "Iq_ref_Spd_loop"
  N_fb/1 -> Sum/2
  N_ref/1 -> Zero_Cancellation/1
  Sum/1 -> Product/2, Discrete PI Controller with anti-windup & reset/1
  Logical Operator/1 -> Discrete PI Controller with anti-windup & reset/4
  Data Store Read1/1 -> AND/1
  Data Store Read2/1 -> AND/2
  AND/1 -> Logical Operator/1
  Zero_Cancellation/1 -> Sum/1
  Kp1/1 -> Product/1, Discrete PI Controller with anti-windup & reset/2
  Data Store Read3/1 -> Sum1/1  "Iq_switch_mem"
  Ki1/1 -> Discrete PI Controller with anti-windup & reset/3
  Product/1 -> Sum1/2
  Sum1/1 -> Discrete PI Controller with anti-windup & reset/5

== system mcb_pmsm_foc_sensorless_f28379d1/Speed Control/SlewRate ==
  Speed_Ref : Inport
  Ramp limiter : Subsystem
  N_ref : Outport
  wires:
  Speed_Ref/1 -> Ramp limiter/1(In1)
  Ramp limiter/1(Out1) -> N_ref/1

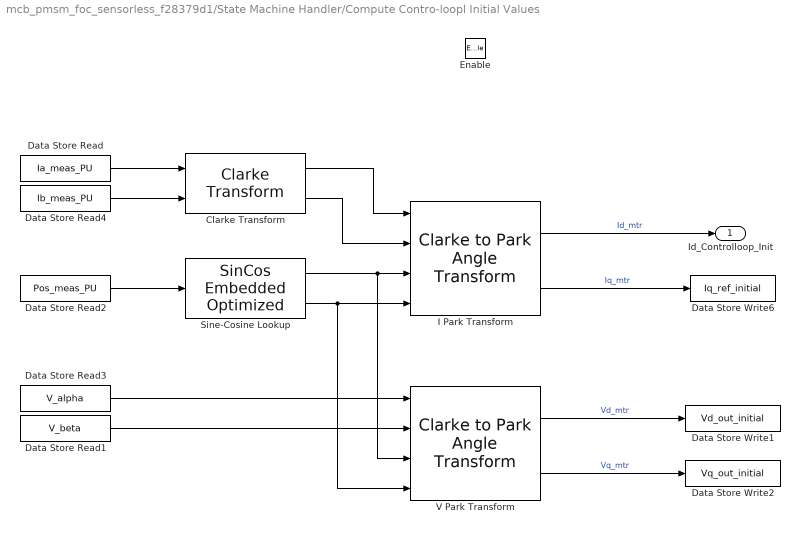
== system mcb_pmsm_foc_sensorless_f28379d1/State Machine Handler/Compute Contro-loopl Initial Values ==
  Enable : EnablePort
  Clarke Transform : mcbeeMathTransformLib/Clarke Transform  VariantControl=Variant2  PowerInvariant=off  UseWithEmbedded=on  PhaseInput=Two inputs
  Data Store Read : DataStoreRead  DataStoreName=Ia_meas_PU  IndexOptions=Index vector (dialog)  Indices=1  OutputSizes=1
  Data Store Read1 : DataStoreRead  DataStoreName=V_beta  IndexOptions=Index vector (dialog)  Indices=1  OutputSizes=1
  Data Store Read2 : DataStoreRead  DataStoreName=Pos_meas_PU  IndexOptions=Index vector (dialog)  Indices=1  OutputSizes=1
  Data Store Read3 : DataStoreRead  DataStoreName=V_alpha  IndexOptions=Index vector (dialog)  Indices=1  OutputSizes=1
  Data Store Read4 : DataStoreRead  DataStoreName=Ib_meas_PU  IndexOptions=Index vector (dialog)  Indices=1  OutputSizes=1
  Data Store Write1 : DataStoreWrite  DataStoreName=Vd_out_initial  IndexOptions=Index vector (dialog)  Indices=1  OutputSizes=1
  Data Store Write2 : DataStoreWrite  DataStoreName=Vq_out_initial  IndexOptions=Index vector (dialog)  Indices=1  OutputSizes=1
  Data Store Write6 : DataStoreWrite  DataStoreName=Iq_ref_initial  IndexOptions=Index vector (dialog)  Indices=1  OutputSizes=1
  I Park Transform : mcbeeMathTransformLib/Clarke to Park Angle Transform  AxisAlignment=D-axis  UseWithEmbedded=on  PhaseInput=Two inputs  ThetaInput=Sine and Cosine electrical position  AngleInput=Per-unit  N_points=1024
  Sine-Cosine Lookup : mcbcontrolslib/SinCos Embedded Optimized  LabelModeActiveChoice=MCB_Sin  OptforProc=off  OptLevelPop=Disabled  ApproximationMethod=None  UserApproxMethod=Lookup  ApproxStatus=None  ThetaDataType=single  CopyThetaDataType=single  InterpMethod=Linear point-slope  NumberOfDataPoints=16  NumberOfIterations=11  RemoveProtectionAgainstOutOfRangeInput=off  TableDataTypeStr=Inherit: Inherit via input  AngleInput=Per-unit  CopyAngleInput=Per-unit  N_points=1024  CopyN_points=1024  Datatype=single  CopyTableDatatype=single  DatatypeInput=Inherit from input  IsPrevStrictOpt=0  IsPrevLUTForced=0
  V Park Transform : mcbeeMathTransformLib/Clarke to Park Angle Transform  AxisAlignment=D-axis  UseWithEmbedded=on  PhaseInput=Two inputs  ThetaInput=Sine and Cosine electrical position  AngleInput=Per-unit  N_points=1024
  Id_Controlloop_Init : Outport
  wires:
  Clarke Transform/1 -> I Park Transform/1
  Sine-Cosine Lookup/1 -> V Park Transform/3, I Park Transform/3
  I Park Transform/1 -> Id_Controlloop_Init/1  "Id_mtr"
  I Park Transform/2 -> Data Store Write6/1  "Iq_mtr"
  Clarke Transform/2 -> I Park Transform/2
  Data Store Read2/1 -> Sine-Cosine Lookup/1
  Sine-Cosine Lookup/2 -> V Park Transform/4, I Park Transform/4
  Data Store Read4/1 -> Clarke Transform/2
  Data Store Read3/1 -> V Park Transform/1
  Data Store Read1/1 -> V Park Transform/2
  V Park Transform/1 -> Data Store Write1/1  "Vd_mtr"
  V Park Transform/2 -> Data Store Write2/1  "Vq_mtr"
  Data Store Read/1 -> Clarke Transform/1

== system mcb_pmsm_foc_sensorless_f28379d1/State Machine Handler/State Machine OL - CL/RunMode.ComputeId0 ==
  Id0_in : Inport  OutDataTypeStr=dataType  PortDimensions=1
  RAMP_STEP_SIZE : Inport  Port=2  OutDataTypeStr=dataType  PortDimensions=1
  f : TriggerPort  TriggerType=function-call  VariantControl=(inherit)
      settings: CopyFcn=Stateflow.SLINSF.SimulinkMan.removeBlockPreDeleteFcn  PreDeleteFcn=Stateflow.SLINSF.SimulinkMan.unsafePredeleteFcn
  Compare To Constant : simulink/Logic and Bit Operations/Compare To Constant  relop=>  const=RAMP_STEP_SIZE  OutDataTypeStr=boolean
  Constant : Constant  Value=0  OutDataTypeStr=Inherit: Inherit via back propagation
  Data Type Duplicate : DataTypeDuplicate
  Sum : Sum  Inputs=+-  RndMeth=Simplest  OutDataTypeStr=Inherit: Same as first input
  Switch : Switch  Criteria=u2 > Threshold  SaturateOnIntegerOverflow=off  InputSameDT=off
  Id0_out : Outport
  wires:
  Id0_in/1 -> Data Type Duplicate/1, Sum/1
  RAMP_STEP_SIZE/1 -> Sum/2
  Sum/1 -> Compare To Constant/1, Switch/1
  Compare To Constant/1 -> Switch/2
  Constant/1 -> Data Type Duplicate/2, Switch/3
  Switch/1 -> Id0_out/1

== system mcb_pmsm_foc_sensorless_f28379d1/Current Control/Closed Loop/Current_Controllers ==
  Id : Inport
  Iq : Inport  Port=2
  Idq_Ref : Inport  Port=3
  DQ Limiter : mcbcontrolslib/DQ Limiter  satMethodInputType=Specify via dialog  satMethodSelected=D-Q equivalence  satLimitInputType=Specify via dialog  Vmax=0.95
  Demux : Demux  Outputs=2
  Mux : Mux
  PI_Controller_Id : Subsystem
  PI_Controller_Iq : Subsystem
  Terminator : Terminator
  Vd_ref : Outport  VectorParamsAs1DForOutWhenUnconnected=off
  Vq_ref : Outport  Port=2  VectorParamsAs1DForOutWhenUnconnected=off
  Idq : Outport  Port=3  VectorParamsAs1DForOutWhenUnconnected=off
  wires:
  Iq/1 -> Mux/4, PI_Controller_Iq/2(I_fb)  "Iq_fb"
  Id/1 -> PI_Controller_Id/2(I_fb), Mux/2  "Id_fb"
  Demux/1 -> PI_Controller_Id/1(I_ref), Mux/1  "Id_Ref"
  Demux/2 -> Mux/3, PI_Controller_Iq/1(I_ref)  "Iq_Ref"
  DQ Limiter/1 -> Vd_ref/1  "Vd_ref"
  DQ Limiter/2 -> Vq_ref/1  "Vq_ref"
  DQ Limiter/3 -> Terminator/1
  Idq_Ref/1 -> Demux/1
  Mux/1 -> Idq/1
  PI_Controller_Id/1(V_ref) -> DQ Limiter/1
  PI_Controller_Iq/1(V_ref) -> DQ Limiter/2

== system mcb_pmsm_foc_sensorless_f28379d1/Current Control/Closed Loop/Open_Loop_Control ==
  Pos_PU : Inport
  Accumulate1 : Subsystem
      settings: LibrarySourceBlock=mcbcontrolslib/Position Generator/Accumulate
  Data Store Read : DataStoreRead  DataStoreName=SpdCtrlRef  IndexOptions=Index vector (dialog)  Indices=1  OutputSizes=1
  Data Store Read1 : DataStoreRead  DataStoreName=EnClosedLoop  IndexOptions=Index vector (dialog)  Indices=1  OutputSizes=1
  Data Store Read2 : DataStoreRead  DataStoreName=EnClosedLoop  IndexOptions=Index vector (dialog)  Indices=1  OutputSizes=1
  Delay : Delay  DelayLength=1  InitialConditionSource=Input port  ExternalReset=Falling
      settings: InputPortMap=u0,r5,p4
  Gain : Gain  Gain=Ts*PU_System.N_base*pmsm.p/60  OutDataTypeStr=Inherit: Same as input  ParamDataTypeStr=Inherit: Same as input
  Position Generator : mcbcontrolslib/Position Generator  AngleOutput=Per-unit  InitialThetaSource=Specify via dialog  ExternalReset=none  Offset=0
  Scope : Scope  NumInputPorts=2
      settings: ActiveDisplayYMinimum=-0.0104  ActiveDisplayYMaximum=1.02306
  Switch : Switch  Criteria=u2 ~= 0  Threshold=0.1  SaturateOnIntegerOverflow=off  InputSameDT=off
  Pos_PU_Out : Outport
  wires:
  Pos_PU/1 -> Delay/3, Switch/1  "SMO_Pos"
  Switch/1 -> Pos_PU_Out/1
  Gain/1 -> Accumulate1/1(Theta), Position Generator/1
  Position Generator/1 -> Scope/1  "Controller_PU"
  Data Store Read/1 -> Gain/1
  Data Store Read1/1 -> Switch/2
  Accumulate1/1(theta_e) -> Delay/1, Switch/3, Scope/2  "Pos_OL"
  Delay/1 -> Accumulate1/2(Theta_e_prev)
  Data Store Read2/1 -> Delay/2

== system mcb_pmsm_foc_sensorless_f28379d1/Current Control/HW_Inputs/Sensor Driver Blocks (codegen) ==
  Sim : Inport
  ADC_B_IN2 : c2802xlib/ADC  blkParamProc=C2000_Type4  ADCModule=B  samplingMode=Single sample mode  ADCResolution=12-bit (Single-ended input)  ADC29xResolution=12-bit  ADCMode=Single-ended input  useSOC1=SOC0  useSOC2=SOC0_SOC1  SOCAcquisitionWindow=15  SOCTriggerSource=ePWM1_ADCSOCA  SOCInterruptTrigger=No ADCINT  Ts=-1  dType=uint16  postInterrupt=on  interruptSel=ADCINT1  ADCINTContinuous=on  endma=off  chdma=1  conv1=ADCINA0  conv2=ADCINA0 and ADCINB0  conv1_Type4=ADCIN2  conv2_Type4=ADCIN0 and ADCIN1
  ADC_C_IN2 : c2802xlib/ADC  blkParamProc=C2000_Type4  ADCModule=C  samplingMode=Single sample mode  ADCResolution=12-bit (Single-ended input)  ADC29xResolution=12-bit  ADCMode=Single-ended input  useSOC1=SOC0  useSOC2=SOC0_SOC1  SOCAcquisitionWindow=15  SOCTriggerSource=ePWM1_ADCSOCA  SOCInterruptTrigger=No ADCINT  Ts=-1  dType=uint16  postInterrupt=off  interruptSel=ADCINT1  ADCINTContinuous=on  endma=off  chdma=1  conv1=ADCINA0  conv2=ADCINA0 and ADCINB0  conv1_Type4=ADCIN2  conv2_Type4=ADCIN0 and ADCIN1
  Mux1 : Mux  Inputs=2
  Terminator : Terminator
  Iab_ADC : Outport
  wires:
  ADC_C_IN2/1 -> Mux1/1
  Mux1/1 -> Iab_ADC/1
  ADC_B_IN2/1 -> Mux1/2
  Sim/1 -> Terminator/1

== system mcb_pmsm_foc_sensorless_f28379d1/Current Control/HW_Inputs/Sensor Driver Blocks (sim) ==
  Sim : Inport
  Iab_ADC : Outport
  wires:
  Sim/1 -> Iab_ADC/1

== system mcb_pmsm_foc_sensorless_f28379d1/Current Control/Input Scaling/Calculate Phase Currents ==
  Iab_ADC : Inport
  Add : Sum  Inputs=-+
  Data Store Read1 : DataStoreRead  DataStoreName=IaOffset  IndexOptions=Index vector (dialog)  Indices=1  OutputSizes=1
  Data Store Read2 : DataStoreRead  DataStoreName=IbOffset  IndexOptions=Index vector (dialog)  Indices=1  OutputSizes=1
  Data Type Conversion : DataTypeConversion  OutDataTypeStr=int32  ConvertRealWorld=Stored Integer (SI)  RndMeth=Simplest  SaturateOnIntegerOverflow=off
  Data_Type : Subsystem  Variant=on
  Inverting / Non-inverting Current measurement amplifier : Gain  Gain=inverter.invertingAmp  RndMeth=Simplest  OutDataTypeStr=Inherit: Same as input
  Mux1 : Mux  Inputs=2
  Iab_meas_PU : Outport  VectorParamsAs1DForOutWhenUnconnected=off
  wires:
  Data Type Conversion/1 -> Add/2
  Add/1 -> Data_Type/1(In1)
  Data_Type/1(Iab_meas_PU) -> Inverting / Non-inverting Current measurement amplifier/1
  Iab_ADC/1 -> Data Type Conversion/1
  Data Store Read1/1 -> Mux1/1
  Data Store Read2/1 -> Mux1/2
  Mux1/1 -> Add/1
  Inverting / Non-inverting Current measurement amplifier/1 -> Iab_meas_PU/1

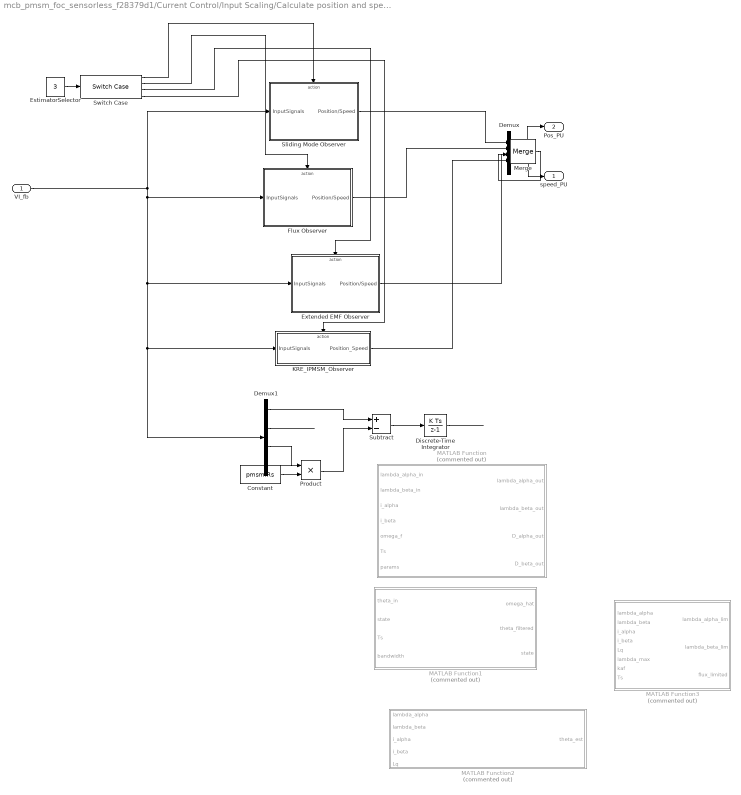
== system mcb_pmsm_foc_sensorless_f28379d1/Current Control/Input Scaling/Calculate position and speed ==
  VI_fb : Inport
  Constant : Constant  Value=pmsm.Rs
  Demux : Demux  Outputs=2
  Demux1 : Demux
  Discrete-Time Integrator : DiscreteIntegrator  SampleTime=-1  ICPrevOutput=DiscIntNeverNeededParam  ICPrevScaledInput=DiscIntNeverNeededParam
  EstimatorSelector : Constant  Value=3  OutDataTypeStr=uint32
  Extended EMF Observer : Subsystem
  Flux Observer : Subsystem
  KRE_IPMSM_Observer : Subsystem
  MATLAB Function : MATLAB Function  Commented=on  TreatAsAtomicUnit=on
  MATLAB Function1 : MATLAB Function  Commented=on  TreatAsAtomicUnit=on
  MATLAB Function2 : MATLAB Function  Commented=on  TreatAsAtomicUnit=on
  MATLAB Function3 : MATLAB Function  Commented=on  TreatAsAtomicUnit=on
  Merge : Merge  Inputs=4
  Product : Product
  Sliding Mode Observer : Subsystem
  Subtract : Sum  Inputs=+-
  Switch Case : SwitchCase  CaseConditions={0,1,2,3}  ShowDefaultCase=off
  speed_PU : Outport
  Pos_PU : Outport  Port=2
  wires:
  Demux/1 -> Pos_PU/1
  Demux/2 -> speed_PU/1
  Demux1/1 -> Subtract/1
  Demux1/2 -> ?
  Demux1/3 -> Product/1
  Demux1/4 -> ?
  Constant/1 -> Product/2
  Product/1 -> Subtract/2
  Subtract/1 -> Discrete-Time Integrator/1
  Discrete-Time Integrator/1 -> ?
  Switch Case/3 -> Extended EMF Observer/Action
  Switch Case/1 -> Sliding Mode Observer/Action
  EstimatorSelector/1 -> Switch Case/1
  KRE_IPMSM_Observer/1(Position_Speed) -> Merge/4
  Sliding Mode Observer/1(Position/Speed) -> Merge/1
  Flux Observer/1(Position/Speed) -> Merge/2
  Merge/1 -> Demux/1
  Switch Case/2 -> Flux Observer/Action
  VI_fb/1 -> Demux1/1, KRE_IPMSM_Observer/1(InputSignals), Extended EMF Observer/1(InputSignals), Flux Observer/1(InputSignals), Sliding Mode Observer/1(InputSignals)
  Extended EMF Observer/1(Position/Speed) -> Merge/3
  Switch Case/4 -> KRE_IPMSM_Observer/Action
